simulink model "maxRadius"  (R2019a)
settings: Solver=VariableStepAuto  StartTime=0.0  StopTime=10.0  RelTol=1e-3
values from neighbouring files (symbols this model uses):
  c_L = 2.85    [Initialisierung.m]
  m = 220    [Initialisierung.m]
  maxV = 110    [Initialisierung.m]
  my = 1.3    [Initialisierung.m]
settings Model: Creator=Frieder Uerlings  LastModifiedBy=Frieder Uerlings

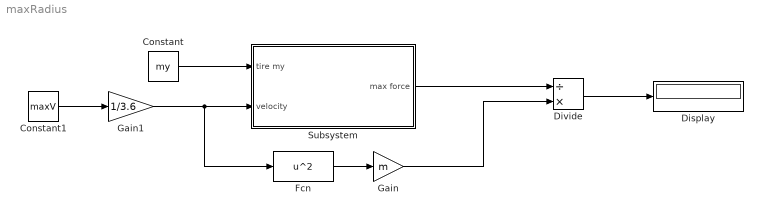
== system maxRadius ==
  Constant : Constant  Value=my
  Constant1 : Constant  Value=maxV
  Display : Display
  Divide : Product  Inputs=/*
  Fcn : Fcn  Expr=u^2
  Gain : Gain  Gain=m
  Gain1 : Gain  Gain=1/3.6
  Subsystem : Subsystem
  wires:
  Gain1/1 -> Fcn/1, Subsystem/2(velocity)
  Constant/1 -> Subsystem/1(tire my)
  Fcn/1 -> Gain/1
  Subsystem/1(max force) -> Divide/1
  Gain/1 -> Divide/2
  Constant1/1 -> Gain1/1
  Divide/1 -> Display/1

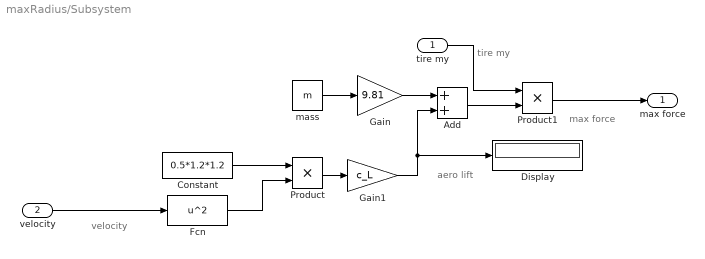
== system maxRadius/Subsystem ==
  note: max force
  note: aero lift
  note: tire my
  note: velocity
  tire my : Inport
  velocity : Inport  Port=2
  Add : Sum
  Constant : Constant  Value=0.5*1.2*1.2
  Display : Display
  Fcn : Fcn  Expr=u^2
  Gain : Gain  Gain=9.81
  Gain1 : Gain  Gain=c_L
  Product : Product
  Product1 : Product
  "mass " : Constant  Value=m
  max force : Outport
  wires:
  Constant/1 -> Product/1
  Add/1 -> Product1/2
  "mass "/1 -> Gain/1
  Fcn/1 -> Product/2
  Product1/1 -> max force/1
  Gain/1 -> Add/1
  Product/1 -> Gain1/1
  tire my/1 -> Product1/1
  velocity/1 -> Fcn/1
  Gain1/1 -> Add/2, Display/1
